simulink model "Pointmass_eom_v1_0"  (R2020a)
settings: Solver=ode4  StartTime=0.0  StopTime=simInit.TSIM  FixedStep=simInit.dt  MaxStep=simInit.dt  RelTol=1e-3
InitFcn:
  | close all
values from neighbouring files (symbols this model uses):
  base_windspeed = 12    [initAllSimParams_DE2019.m]
undefined symbols (not defined in the file or in its folder): constr, DE2019, DiscIntNeverNeededParam, ENVMT, Lbooth, loiterStates, params, simInit, T
libraries: simulink x26, simulink_extras x3
(part 2 of 4)

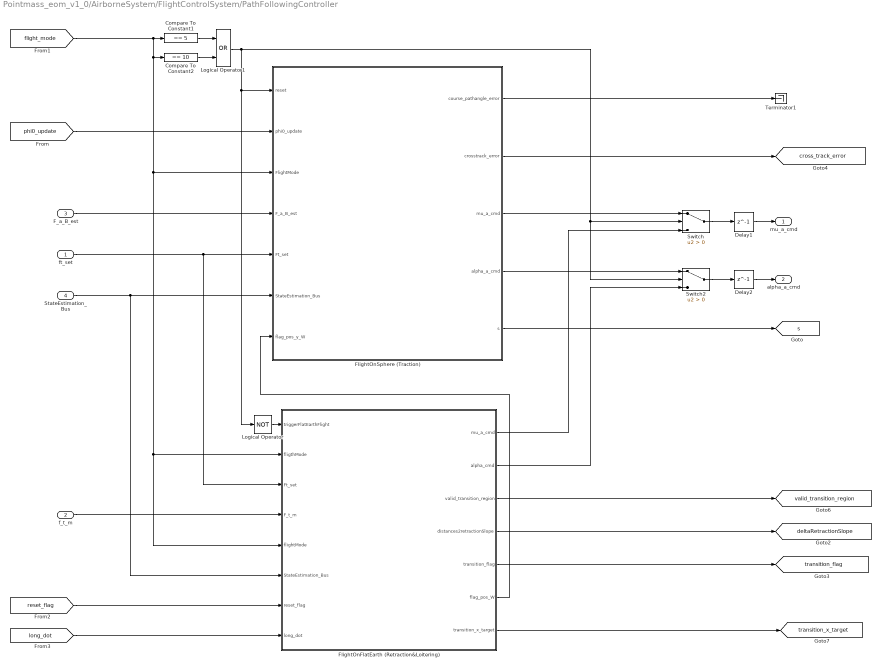
== system Pointmass_eom_v1_0/AirborneSystem/FlightControlSystem/PathFollowingController ==
  ft_set : Inport
  f_t_m : Inport  Port=2
  F_a_B_est : Inport  Port=3  PortDimensions=[3,1]
  StateEstimation_Bus : Inport  Port=4
  Compare To Constant1 : simulink/Logic and Bit Operations/Compare To Constant  relop===  const=5  OutDataTypeStr=boolean
  Compare To Constant2 : simulink/Logic and Bit Operations/Compare To Constant  relop===  const=10  OutDataTypeStr=boolean
  Delay1 : Delay  DelayLength=1
  Delay2 : Delay  DelayLength=1
  FlightOnFlatEarth (Retraction&Loitering) : Subsystem
  FlightOnSphere (Traction) : Subsystem
  Logical Operator : Logic  Operator=NOT  AllPortsSameDT=off  OutDataTypeStr=boolean
  Logical Operator1 : Logic  Operator=OR  AllPortsSameDT=off  OutDataTypeStr=boolean
  Switch : Switch  Criteria=u2 > Threshold
  Switch2 : Switch  Criteria=u2 > Threshold
  Terminator1 : Terminator
  mu_a_cmd : Outport  PortDimensions=1  VectorParamsAs1DForOutWhenUnconnected=off
  alpha_a_cmd : Outport  Port=2  PortDimensions=1  VectorParamsAs1DForOutWhenUnconnected=off
  tag scope: cross_track_error=global, deltaRetractionSlope=global, s=global, transition_flag=global, transition_x_target=global, valid_transition_region=global
  wires:
  StateEstimation_Bus/1 -> FlightOnFlatEarth (Retraction&Loitering)/6(StateEstimation_Bus), FlightOnSphere (Traction)/6(StateEstimation_Bus)
  Logical Operator1/1 -> Switch2/2, Switch/2, FlightOnSphere (Traction)/1(reset), Logical Operator/1
  FlightOnFlatEarth (Retraction&Loitering)/3(valid_transition_region) -> [valid_transition_region]
  FlightOnFlatEarth (Retraction&Loitering)/2(alpha_cmd) -> Switch2/3
  FlightOnFlatEarth (Retraction&Loitering)/1(mu_a_cmd) -> Switch/3
  Logical Operator/1 -> FlightOnFlatEarth (Retraction&Loitering)/1(triggerFlatEarthFlight)
  ft_set/1 -> FlightOnFlatEarth (Retraction&Loitering)/3(Ft_set), FlightOnSphere (Traction)/5(Ft_set)
  Delay2/1 -> alpha_a_cmd/1
  Delay1/1 -> mu_a_cmd/1
  Switch/1 -> Delay1/1
  Switch2/1 -> Delay2/1
  f_t_m/1 -> FlightOnFlatEarth (Retraction&Loitering)/4(F_t_m)
  F_a_B_est/1 -> FlightOnSphere (Traction)/4(F_a_B_est)
  FlightOnSphere (Traction)/4(alpha_a_cmd) -> Switch2/1
  FlightOnSphere (Traction)/3(mu_a_cmd) -> Switch/1
  FlightOnSphere (Traction)/1(course_pathangle_error) -> Terminator1/1
  FlightOnSphere (Traction)/2(crosstrack_error) -> [cross_track_error]
  [flight_mode] -> FlightOnFlatEarth (Retraction&Loitering)/5(flightMode), FlightOnFlatEarth (Retraction&Loitering)/2(fligthMode), FlightOnSphere (Traction)/3(FlightMode), Compare To Constant2/1, Compare To Constant1/1
  Compare To Constant1/1 -> Logical Operator1/1
  Compare To Constant2/1 -> Logical Operator1/2
  FlightOnSphere (Traction)/5(s) -> [s]
  [phi0_update] -> FlightOnSphere (Traction)/2(phi0_update)
  FlightOnFlatEarth (Retraction&Loitering)/5(transition_flag) -> [transition_flag]
  [reset_flag] -> FlightOnFlatEarth (Retraction&Loitering)/7(reset_flag)
  FlightOnFlatEarth (Retraction&Loitering)/4(distances2retractionSlope) -> [deltaRetractionSlope]
  FlightOnFlatEarth (Retraction&Loitering)/6(flag_pos_W) -> FlightOnSphere (Traction)/7(flag_pos_y_W)
  [long_dot] -> FlightOnFlatEarth (Retraction&Loitering)/8(long_dot)
  FlightOnFlatEarth (Retraction&Loitering)/7(transition_x_target) -> [transition_x_target]

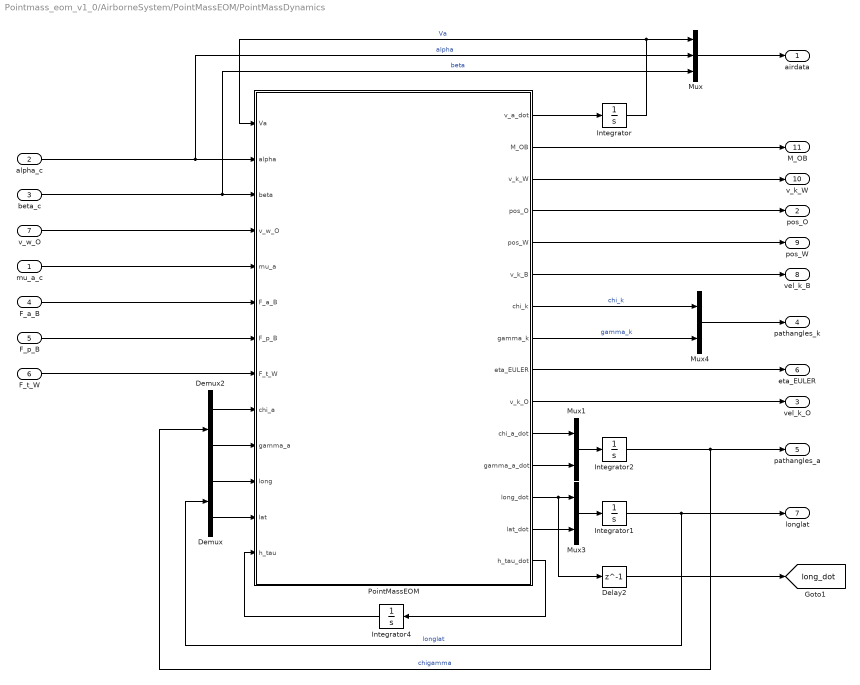
== system Pointmass_eom_v1_0/AirborneSystem/PointMassEOM/PointMassDynamics ==
  mu_a_c : Inport
  alpha_c : Inport  Port=2
  beta_c : Inport  Port=3
  F_a_B : Inport  Port=4  PortDimensions=[3,1]
  F_p_B : Inport  Port=5  PortDimensions=[3,1]
  F_t_W : Inport  Port=6  PortDimensions=[3,1]
  v_w_O : Inport  Port=7
  Delay2 : Delay  DelayLength=1
  Demux : Demux  Outputs=2
  Demux2 : Demux  Outputs=2
  Integrator : Integrator  InitialCondition=.7*loiterStates.Va_set
  Integrator1 : Integrator  InitialCondition=[simInit.long_init;simInit.lat_init]  WrapState=on
  Integrator2 : Integrator  WrapState=on
  Integrator4 : Integrator  InitialCondition=norm(simInit.pos_O_init)
  Mux : Mux  Inputs=3
  Mux1 : Mux  Inputs=2
  Mux3 : Mux  Inputs=2
  Mux4 : Mux  Inputs=2
  PointMassEOM : MATLAB Function  TreatAsAtomicUnit=on
  airdata : Outport  PortDimensions=3  VectorParamsAs1DForOutWhenUnconnected=off
  pos_O : Outport  Port=2  PortDimensions=[3,1]  VectorParamsAs1DForOutWhenUnconnected=off
  vel_k_O : Outport  Port=3  PortDimensions=[3,1]  VectorParamsAs1DForOutWhenUnconnected=off
  pathangles_k : Outport  Port=4  PortDimensions=2  VectorParamsAs1DForOutWhenUnconnected=off
  pathangles_a : Outport  Port=5  PortDimensions=2  VectorParamsAs1DForOutWhenUnconnected=off
  eta_EULER : Outport  Port=6  PortDimensions=[3,1]  VectorParamsAs1DForOutWhenUnconnected=off
  longlat : Outport  Port=7  PortDimensions=2  VectorParamsAs1DForOutWhenUnconnected=off
  vel_k_B : Outport  Port=8  PortDimensions=[3,1]  VectorParamsAs1DForOutWhenUnconnected=off
  pos_W : Outport  Port=9  PortDimensions=[3,1]  VectorParamsAs1DForOutWhenUnconnected=off
  v_k_W : Outport  Port=10  PortDimensions=[3,1]  VectorParamsAs1DForOutWhenUnconnected=off
  M_OB : Outport  Port=11  PortDimensions=[3,3]  VectorParamsAs1DForOutWhenUnconnected=off
  tag scope: long_dot=global
  wires:
  F_p_B/1 -> PointMassEOM/7(F_p_B)
  mu_a_c/1 -> PointMassEOM/5(mu_a)
  PointMassEOM/7(chi_k) -> Mux4/1  "chi_k"
  F_a_B/1 -> PointMassEOM/6(F_a_B)
  Integrator/1 -> PointMassEOM/1(Va), Mux/1  "Va"
  PointMassEOM/8(gamma_k) -> Mux4/2  "gamma_k"
  PointMassEOM/12(gamma_a_dot) -> Mux1/2
  Integrator4/1 -> PointMassEOM/13(h_tau)
  PointMassEOM/14(lat_dot) -> Mux3/2
  PointMassEOM/11(chi_a_dot) -> Mux1/1
  PointMassEOM/15(h_tau_dot) -> Integrator4/1
  PointMassEOM/1(v_a_dot) -> Integrator/1
  Demux2/2 -> PointMassEOM/10(gamma_a)
  v_w_O/1 -> PointMassEOM/4(v_w_O)
  PointMassEOM/9(eta_EULER) -> eta_EULER/1
  Mux/1 -> airdata/1
  alpha_c/1 -> PointMassEOM/2(alpha), Mux/2  "alpha"
  beta_c/1 -> Mux/3, PointMassEOM/3(beta)  "beta"
  PointMassEOM/10(v_k_O) -> vel_k_O/1
  PointMassEOM/6(v_k_B) -> vel_k_B/1
  PointMassEOM/5(pos_W) -> pos_W/1
  PointMassEOM/4(pos_O) -> pos_O/1
  Mux4/1 -> pathangles_k/1
  Demux2/1 -> PointMassEOM/9(chi_a)
  PointMassEOM/3(v_k_W) -> v_k_W/1
  PointMassEOM/2(M_OB) -> M_OB/1
  PointMassEOM/13(long_dot) -> Mux3/1, Delay2/1
  Mux3/1 -> Integrator1/1
  Delay2/1 -> [long_dot]
  Integrator1/1 -> longlat/1, Demux/1  "longlat"
  Demux/1 -> PointMassEOM/11(long)
  Demux/2 -> PointMassEOM/12(lat)
  Mux1/1 -> Integrator2/1
  Integrator2/1 -> pathangles_a/1, Demux2/1  "chigamma"
  F_t_W/1 -> PointMassEOM/8(F_t_W)

== system Pointmass_eom_v1_0/Environment/ShearWind/Length Conversion ==
  in : Inport  Unit=m
  Unit Conversion : UnitConversion
  out : Outport  Unit=ft  VectorParamsAs1DForOutWhenUnconnected=off
  wires:
  in/1 -> Unit Conversion/1
  Unit Conversion/1 -> out/1

== system Pointmass_eom_v1_0/Environment/Windshear/Wind Shear Model ==
  Altitude : Inport  Unit=m
  DCM : Inport  Port=2  Unit=1  PortDimensions=[3 3]
  3ft-->inf1 : Saturate  UpperLimit=inf  LowerLimit=3
  Degrees to Radians : simulink_extras/Transformations/Degrees to Radians
  Disallow CGS : UnitConfiguration  UnitSystemsStr=English,SI,SI (extended)  AllowAllUnitSystems=off
  Length Conversion1 : Subsystem
  Mux : Mux  Inputs=3
  Product2 : Product  Inputs=*/  InputSameDT=on  SaturateOnIntegerOverflow=on  OutDataTypeStr=Inherit: Same as first input
  Product3 : Product  InputSameDT=on  SaturateOnIntegerOverflow=on  OutDataTypeStr=Inherit: Same as first input
  Reshape : Reshape  OutputDimensionality=Column vector (2-D)
  Reshape1 : Reshape
  SinCos : Trigonometry  Operator=sincos
  Transform from Inertial to Body axes : Product  Inputs=**  Multiplication=Matrix(*)  InputSameDT=on  SaturateOnIntegerOverflow=on  OutDataTypeStr=Inherit: Same as first input
  Wdeg1 : Constant  Value=0  OutDataTypeStr=Inherit: Inherit via back propagation
  Wind Direction : Constant  Value=ENVMT.windDirection_rad*180/pi  OutDataTypeStr=Inherit: Inherit via back propagation
  Wind speed at reference height : Gain  Gain=-base_windspeed  SaturateOnIntegerOverflow=on  OutDataTypeStr=Inherit: Same as input  ParamDataTypeStr=Inherit: Same as input
  h/z1 : Gain  Gain=1/0.15  SaturateOnIntegerOverflow=on  OutDataTypeStr=Inherit: Same as input  ParamDataTypeStr=Inherit: Same as input
  ln(h/z0)1 : Math  Operator=log  SignedPower=on  SaturateOnIntegerOverflow=on
  ln(ref_height/z0)1 : Math  Operator=log  SignedPower=on  SaturateOnIntegerOverflow=on
  ref_height/z0 [ft] : Constant  Value=20/0.15  OutDataTypeStr=Inherit: Inherit via back propagation
  Mean Wind : Outport  Unit=m/s  VectorParamsAs1DForOutWhenUnconnected=off
  wires:
  Reshape1/1 -> Mean Wind/1
  Reshape/1 -> Transform from Inertial to Body axes/2
  Degrees to Radians/1 -> SinCos/1
  Wind speed at reference height/1 -> Product3/2
  DCM/1 -> Transform from Inertial to Body axes/1
  Product3/1 -> Reshape/1
  Mux/1 -> Wind speed at reference height/1
  Wdeg1/1 -> Mux/3  "Wz"
  SinCos/1 -> Mux/2  "Wy"
  SinCos/2 -> Mux/1  "Wx"
  Wind Direction/1 -> Degrees to Radians/1
  Transform from Inertial to Body axes/1 -> Reshape1/1
  Altitude/1 -> Length Conversion1/1(in)
  Length Conversion1/1(out) -> 3ft-->inf1/1
  ln(h/z0)1/1 -> Product2/1
  ln(ref_height/z0)1/1 -> Product2/2
  Product2/1 -> Product3/1
  3ft-->inf1/1 -> h/z1/1
  ref_height/z0 [ft]/1 -> ln(ref_height/z0)1/1
  h/z1/1 -> ln(h/z0)1/1

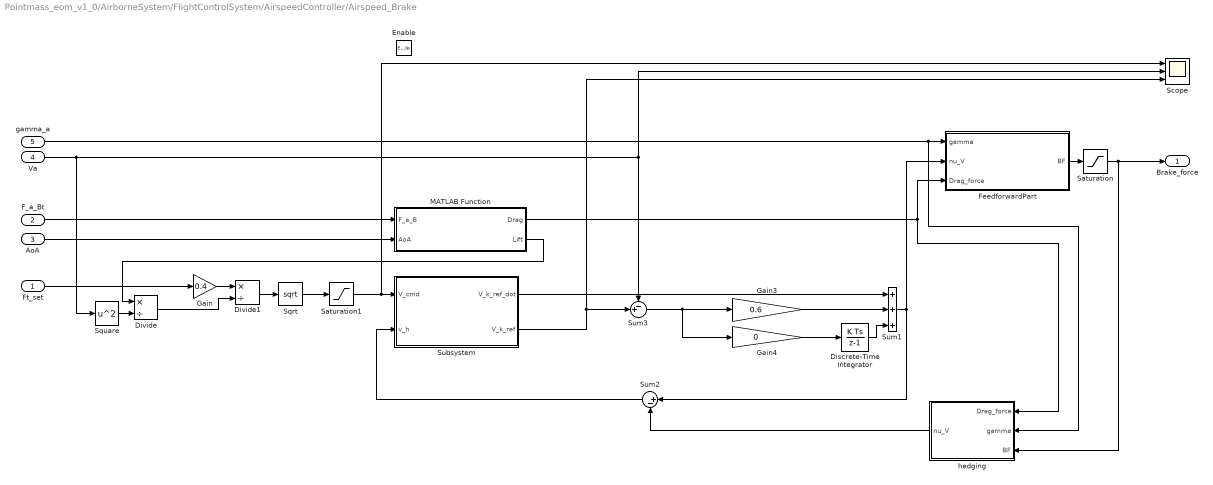
== system Pointmass_eom_v1_0/AirborneSystem/FlightControlSystem/AirspeedController/Airspeed_Brake ==
  Ft_set : Inport
  F_a_Bt : Inport  Port=2  PortDimensions=[3,1]
  AoA : Inport  Port=3
  Va : Inport  Port=4
  gamma_a : Inport  Port=5
  Enable : EnablePort
  Discrete-Time Integrator : DiscreteIntegrator  SampleTime=-1  ICPrevOutput=DiscIntNeverNeededParam  ICPrevScaledInput=DiscIntNeverNeededParam
  Divide : Product  Inputs=*/
  Divide1 : Product  Inputs=*/
  FeedforwardPart : MATLAB Function  TreatAsAtomicUnit=on
  Gain : Gain  Gain=0.4
  Gain3 : Gain  Gain=0.6
  Gain4 : Gain  Gain=0
  MATLAB Function : MATLAB Function  TreatAsAtomicUnit=on
  Saturation : Saturate  UpperLimit=0  LowerLimit=-inf  LinearizeAsGain=off
  Saturation1 : Saturate  UpperLimit=inf  LowerLimit=35
  Scope : Scope  NumInputPorts=3
  Sqrt : Sqrt  SaturateOnIntegerOverflow=on
  Square : Math  Operator=square  SaturateOnIntegerOverflow=on
  Subsystem : Subsystem
  Sum1 : Sum  Inputs=+++
  Sum2 : Sum  Inputs=|+-
  Sum3 : Sum  Inputs=-+|
  hedging : MATLAB Function  TreatAsAtomicUnit=on
  Brake_force : Outport  VectorParamsAs1DForOutWhenUnconnected=off
  wires:
  AoA/1 -> MATLAB Function/2(AoA)
  MATLAB Function/1(Drag) -> hedging/1(Drag_force), FeedforwardPart/3(Drag_force)
  F_a_Bt/1 -> MATLAB Function/1(F_a_B)
  Sum2/1 -> Subsystem/2(v_h)
  hedging/1(nu_V) -> Sum2/2
  FeedforwardPart/1(BF) -> Saturation/1
  Saturation/1 -> hedging/3(BF), Brake_force/1
  Subsystem/1(V_k_ref_dot) -> Sum1/1
  Sum1/1 -> FeedforwardPart/2(nu_V), Sum2/1
  Subsystem/2(V_k_ref) -> Sum3/2, Scope/3
  gamma_a/1 -> hedging/2(gamma), FeedforwardPart/1(gamma)
  Sqrt/1 -> Saturation1/1
  Sum3/1 -> Gain4/1, Gain3/1
  Gain3/1 -> Sum1/2
  Discrete-Time Integrator/1 -> Sum1/3
  Gain4/1 -> Discrete-Time Integrator/1
  MATLAB Function/2(Lift) -> Divide/1
  Va/1 -> Sum3/1, Scope/2, Square/1
  Square/1 -> Divide/2
  Ft_set/1 -> Gain/1
  Divide/1 -> Divide1/2
  Divide1/1 -> Sqrt/1
  Gain/1 -> Divide1/1
  Saturation1/1 -> Subsystem/1(V_cmd), Scope/1

== system Pointmass_eom_v1_0/AirborneSystem/FlightControlSystem/AirspeedController/Airspeed_Control ==
  V_CMD : Inport
  F_a_B : Inport  Port=2  PortDimensions=[3,1]
  AoA : Inport  Port=3
  Va : Inport  Port=4
  gamma_a : Inport  Port=5
  Enable : EnablePort
  Discrete-Time Integrator : DiscreteIntegrator  SampleTime=-1  ICPrevOutput=DiscIntNeverNeededParam  ICPrevScaledInput=DiscIntNeverNeededParam
  FeedforwardPart : MATLAB Function  TreatAsAtomicUnit=on
  Gain3 : Gain  Gain=params.kp_speed_control
  Gain4 : Gain  Gain=params.ki_speed_control
  MATLAB Function : MATLAB Function  TreatAsAtomicUnit=on
  Saturation : Saturate  UpperLimit=inf  LowerLimit=0  LinearizeAsGain=off
  Scope : Scope  NumInputPorts=3
  Subsystem : Subsystem
  Sum : Sum  Inputs=-+|
  Sum1 : Sum  Inputs=+++
  Sum2 : Sum  Inputs=|+-
  hedging : MATLAB Function  TreatAsAtomicUnit=on
  thrust_force : Outport  VectorParamsAs1DForOutWhenUnconnected=off
  wires:
  AoA/1 -> MATLAB Function/2(AoA)
  MATLAB Function/1(Drag) -> hedging/1(Drag_force), FeedforwardPart/3(Drag_force)
  F_a_B/1 -> MATLAB Function/1(F_a_B)
  Sum2/1 -> Subsystem/2(v_h)
  hedging/1(nu_V) -> Sum2/2
  FeedforwardPart/1(T) -> Saturation/1
  Saturation/1 -> thrust_force/1, hedging/3(T)
  Subsystem/1(V_k_ref_dot) -> Sum1/1
  Sum1/1 -> Sum2/1, FeedforwardPart/2(nu_V)
  Subsystem/2(V_k_ref) -> Sum/2, Scope/3
  gamma_a/1 -> hedging/2(gamma), FeedforwardPart/1(gamma)
  V_CMD/1 -> Subsystem/1(V_cmd), Scope/1
  Sum/1 -> Gain4/1, Gain3/1
  Va/1 -> Scope/2, Sum/1
  Gain3/1 -> Sum1/2
  Discrete-Time Integrator/1 -> Sum1/3
  Gain4/1 -> Discrete-Time Integrator/1

== system Pointmass_eom_v1_0/AirborneSystem/FlightControlSystem/PathFollowingController/FlightOnFlatEarth (Retraction&Loitering) ==
  triggerFlatEarthFlight : Inport
  fligthMode : Inport  Port=2
  Ft_set : Inport  Port=3
  F_t_m : Inport  Port=4
  flightMode : Inport  Port=5
  StateEstimation_Bus : Inport  Port=6
  reset_flag : Inport  Port=7
  long_dot : Inport  Port=8
  CalculateAttitudeCmds : Subsystem
  GuidanceFlatEarth : Subsystem
  mu_a_cmd : Outport  VectorParamsAs1DForOutWhenUnconnected=off
  alpha_cmd : Outport  Port=2  VectorParamsAs1DForOutWhenUnconnected=off
  valid_transition_region : Outport  Port=3  VectorParamsAs1DForOutWhenUnconnected=off
  distances2retractionSlope : Outport  Port=4  VectorParamsAs1DForOutWhenUnconnected=off
  transition_flag : Outport  Port=5  VectorParamsAs1DForOutWhenUnconnected=off
  flag_pos_W : Outport  Port=6  VectorParamsAs1DForOutWhenUnconnected=off
  transition_x_target : Outport  Port=7  VectorParamsAs1DForOutWhenUnconnected=off
  wires:
  StateEstimation_Bus/1 -> GuidanceFlatEarth/2(StateEstimation_Bus), CalculateAttitudeCmds/6(StateEstimation_Bus)
  CalculateAttitudeCmds/1(mu_a_cmd) -> mu_a_cmd/1
  Ft_set/1 -> CalculateAttitudeCmds/3(Ft_set)
  CalculateAttitudeCmds/2(alpha_cmd) -> alpha_cmd/1
  fligthMode/1 -> GuidanceFlatEarth/1(flightMode)
  triggerFlatEarthFlight/1 -> GuidanceFlatEarth/Enable, CalculateAttitudeCmds/1(flight_on_flatearth_flag)
  GuidanceFlatEarth/2(valid_transition_region) -> valid_transition_region/1
  F_t_m/1 -> CalculateAttitudeCmds/4(F_t_m)
  GuidanceFlatEarth/1(distances2slope) -> distances2retractionSlope/1
  GuidanceFlatEarth/3(course_path) -> CalculateAttitudeCmds/2(pathangles_k_cmd)
  flightMode/1 -> CalculateAttitudeCmds/5(flightMode)
  GuidanceFlatEarth/4(transition_flag) -> transition_flag/1
  reset_flag/1 -> GuidanceFlatEarth/3(reset_flat)
  GuidanceFlatEarth/5(flag_pos_W) -> flag_pos_W/1
  long_dot/1 -> GuidanceFlatEarth/4(long_dot)
  GuidanceFlatEarth/6(transition_x_target) -> transition_x_target/1

== system Pointmass_eom_v1_0/AirborneSystem/FlightControlSystem/PathFollowingController/FlightOnSphere (Traction) ==
  reset : Inport
  phi0_update : Inport  Port=2
  FlightMode : Inport  Port=3  PortDimensions=1
  F_a_B_est : Inport  Port=4  PortDimensions=[3,1]
  Ft_set : Inport  Port=5
  StateEstimation_Bus : Inport  Port=6
  flag_pos_y_W : Inport  Port=7
  Constant : Constant  Value=Lbooth.init_sol
  FlightPathLoopTraction : Subsystem
  Navigator : Subsystem
  Pcontroller_ChiGamma_Traction : Subsystem
  Select_init_sol_for_pathfollowing : Stateflow chart  TreatAsAtomicUnit=on
  Sum : Sum  Inputs=|++
  Sum1 : Sum  Inputs=|++
  course_pathangle_error : Outport  VectorParamsAs1DForOutWhenUnconnected=off
  crosstrack_error : Outport  Port=2  VectorParamsAs1DForOutWhenUnconnected=off
  mu_a_cmd : Outport  Port=3  PortDimensions=1  VectorParamsAs1DForOutWhenUnconnected=off
  alpha_a_cmd : Outport  Port=4  PortDimensions=1  VectorParamsAs1DForOutWhenUnconnected=off
  s : Outport  Port=5  VectorParamsAs1DForOutWhenUnconnected=off
  wires:
  FlightPathLoopTraction/1(mu_a_c_traction) -> mu_a_cmd/1
  Navigator/5(course_pathangle_error) -> Pcontroller_ChiGamma_Traction/1(course_pathangle_error), course_pathangle_error/1
  Navigator/1(crosstrack_error) -> crosstrack_error/1
  FlightPathLoopTraction/2(alpha_rq) -> alpha_a_cmd/1
  F_a_B_est/1 -> FlightPathLoopTraction/2(F_a_B_est)
  Ft_set/1 -> FlightPathLoopTraction/1(Ft_set)
  StateEstimation_Bus/1 -> FlightPathLoopTraction/3(StateEstimation_Bus), Navigator/3(StateEstimation_Bus)
  Navigator/2(s) -> s/1
  phi0_update/1 -> Navigator/1(phi0_update)
  reset/1 -> FlightPathLoopTraction/Enable, Navigator/Enable
  Navigator/3(chi_k_dot) -> Sum/1
  Navigator/4(gamma_k_dot) -> Sum1/1
  Select_init_sol_for_pathfollowing/1(sol_init) -> Navigator/4(init_value)
  Constant/1 -> Select_init_sol_for_pathfollowing/1(x)
  Sum1/1 -> FlightPathLoopTraction/5(nu_gamma)
  Sum/1 -> FlightPathLoopTraction/4(nu_chi)
  FlightMode/1 -> Navigator/2(flight_mode), Select_init_sol_for_pathfollowing/2(fm)
  flag_pos_y_W/1 -> Select_init_sol_for_pathfollowing/3(flag_pos_y_W)
  Pcontroller_ChiGamma_Traction/1(Chi_cntr) -> Sum/2
  Pcontroller_ChiGamma_Traction/2(Gamma_cntr) -> Sum1/2

== system Pointmass_eom_v1_0/Environment/Windshear/Wind Shear Model/Length Conversion1 ==
  in : Inport  Unit=m
  Unit Conversion : UnitConversion
  out : Outport  Unit=ft  VectorParamsAs1DForOutWhenUnconnected=off
  wires:
  in/1 -> Unit Conversion/1
  Unit Conversion/1 -> out/1

== system Pointmass_eom_v1_0/AirborneSystem/FlightControlSystem/AirspeedController/Airspeed_Brake/Subsystem ==
  V_cmd : Inport
  v_h : Inport  Port=2
  Discrete-Time Integrator1 : DiscreteIntegrator  InitialCondition=norm(simInit.vel_B_init)  SampleTime=-1  LimitOutput=on  UpperSaturationLimit=120  LowerSaturationLimit=0  ICPrevOutput=DiscIntNeverNeededParam  ICPrevScaledInput=DiscIntNeverNeededParam
  Gain2 : Gain  Gain=params.w0SpeedControl  Multiplication=Matrix(K*u)
  Sum1 : Sum  Inputs=|+-
  Sum2 : Sum  Inputs=|+-
  V_k_ref_dot : Outport  VectorParamsAs1DForOutWhenUnconnected=off
  V_k_ref : Outport  Port=2  VectorParamsAs1DForOutWhenUnconnected=off
  wires:
  Gain2/1 -> Sum1/1, V_k_ref_dot/1
  v_h/1 -> Sum1/2
  Sum1/1 -> Discrete-Time Integrator1/1
  V_cmd/1 -> Sum2/1
  Sum2/1 -> Gain2/1
  Discrete-Time Integrator1/1 -> V_k_ref/1, Sum2/2

== system Pointmass_eom_v1_0/AirborneSystem/FlightControlSystem/AirspeedController/Airspeed_Control/Subsystem ==
  V_cmd : Inport
  v_h : Inport  Port=2
  Discrete-Time Integrator1 : DiscreteIntegrator  InitialCondition=norm(simInit.vel_B_init)  SampleTime=-1  LimitOutput=on  UpperSaturationLimit=120  LowerSaturationLimit=0  ICPrevOutput=DiscIntNeverNeededParam  ICPrevScaledInput=DiscIntNeverNeededParam
  Gain2 : Gain  Gain=params.w0SpeedControl  Multiplication=Matrix(K*u)
  Sum1 : Sum  Inputs=|+-
  Sum2 : Sum  Inputs=|+-
  V_k_ref_dot : Outport  VectorParamsAs1DForOutWhenUnconnected=off
  V_k_ref : Outport  Port=2  VectorParamsAs1DForOutWhenUnconnected=off
  wires:
  Gain2/1 -> Sum1/1, V_k_ref_dot/1
  v_h/1 -> Sum1/2
  Sum1/1 -> Discrete-Time Integrator1/1
  V_cmd/1 -> Sum2/1
  Sum2/1 -> Gain2/1
  Discrete-Time Integrator1/1 -> V_k_ref/1, Sum2/2

== system Pointmass_eom_v1_0/AirborneSystem/FlightControlSystem/PathFollowingController/FlightOnFlatEarth (Retraction&Loitering)/CalculateAttitudeCmds ==
  flight_on_flatearth_flag : Inport
  pathangles_k_cmd : Inport  Port=2
  Ft_set : Inport  Port=3
  F_t_m : Inport  Port=4
  flightMode : Inport  Port=5
  StateEstimation_Bus : Inport  Port=6
  Demux : Demux  Outputs=3
  FlightPathLoopRetraction_Aerodynamic : Subsystem
  Mux1 : Mux  Inputs=3
  Signal Specification : SignalSpecification  Dimensions=[3,1]
  Terminator2 : Terminator
  mu_a_cmd : Outport  VectorParamsAs1DForOutWhenUnconnected=off
  alpha_cmd : Outport  Port=2  VectorParamsAs1DForOutWhenUnconnected=off
  wires:
  StateEstimation_Bus/1 -> FlightPathLoopRetraction_Aerodynamic/4(StateEstimation_Bus)
  Demux/3 -> Terminator2/1
  Demux/2 -> alpha_cmd/1
  flight_on_flatearth_flag/1 -> FlightPathLoopRetraction_Aerodynamic/Enable
  FlightPathLoopRetraction_Aerodynamic/2(alpha_a_cmd) -> Mux1/2
  flightMode/1 -> FlightPathLoopRetraction_Aerodynamic/1(flight_mode)
  Signal Specification/1 -> Demux/1
  Demux/1 -> mu_a_cmd/1
  Mux1/1 -> Signal Specification/1
  F_t_m/1 -> FlightPathLoopRetraction_Aerodynamic/3(F_t_m)
  FlightPathLoopRetraction_Aerodynamic/1(mu_a_cmd) -> Mux1/1
  Ft_set/1 -> FlightPathLoopRetraction_Aerodynamic/2(F_t_set)
  FlightPathLoopRetraction_Aerodynamic/3(beta_a_cmd) -> Mux1/3
  pathangles_k_cmd/1 -> FlightPathLoopRetraction_Aerodynamic/5(kinematic_path_cmd)

== system Pointmass_eom_v1_0/AirborneSystem/FlightControlSystem/PathFollowingController/FlightOnFlatEarth (Retraction&Loitering)/GuidanceFlatEarth ==
  flightMode : Inport
  StateEstimation_Bus : Inport  Port=2
  reset_flat : Inport  Port=3
  long_dot : Inport  Port=4
  Enable : EnablePort
  Bus Selector : BusSelector  OutputSignals=pos_G_O_m,vel_K_O_mDs,pathangles_k,pos_G_W
  Compare To Constant : simulink/Logic and Bit Operations/Compare To Constant  relop===  const=6  OutDataTypeStr=boolean
  Compare To Constant2 : simulink/Logic and Bit Operations/Compare To Constant  relop===  const=6  OutDataTypeStr=boolean
  LoiteringGuidance : Subsystem
  Retraction_Nav : Subsystem
  Switch1 : Switch  Criteria=u2 > Threshold
  distances2slope : Outport  VectorParamsAs1DForOutWhenUnconnected=off
  valid_transition_region : Outport  Port=2  VectorParamsAs1DForOutWhenUnconnected=off
  course_path : Outport  Port=3  VectorParamsAs1DForOutWhenUnconnected=off
  transition_flag : Outport  Port=4  VectorParamsAs1DForOutWhenUnconnected=off
  flag_pos_W : Outport  Port=5  VectorParamsAs1DForOutWhenUnconnected=off
  transition_x_target : Outport  Port=6  VectorParamsAs1DForOutWhenUnconnected=off
  wires:
  Bus Selector/1 -> LoiteringGuidance/2(<pos_G_O_m>), Retraction_Nav/2(pos_O)  "<pos_G_O_m>"
  StateEstimation_Bus/1 -> Bus Selector/1
  Bus Selector/2 -> LoiteringGuidance/3(<vel_K_O_mDs>), Retraction_Nav/3(vel_k_O)  "<vel_K_O_mDs>"
  Compare To Constant2/1 -> Retraction_Nav/Enable
  Switch1/1 -> course_path/1
  Compare To Constant/1 -> Switch1/2
  Retraction_Nav/1(distances2slope) -> distances2slope/1
  Retraction_Nav/2(path_k_cmds) -> Switch1/1
  flightMode/1 -> Retraction_Nav/1(flight_mode), Compare To Constant/1, LoiteringGuidance/1(flightMode), Compare To Constant2/1
  Bus Selector/3 -> LoiteringGuidance/4(<pathangles_k>)  "<pathangles_k>"
  LoiteringGuidance/1(path_k_cmds) -> Switch1/3
  LoiteringGuidance/2(valid_transition_region) -> valid_transition_region/1
  Retraction_Nav/3(transition_flag) -> transition_flag/1
  reset_flat/1 -> LoiteringGuidance/6(reset_flag)
  Bus Selector/4 -> LoiteringGuidance/5(pos_W)  "<pos_G_W>"
  Retraction_Nav/4(flag_pos_y_W) -> flag_pos_W/1
  long_dot/1 -> Retraction_Nav/4(long_dot)
  Retraction_Nav/5(transition_x_target) -> transition_x_target/1

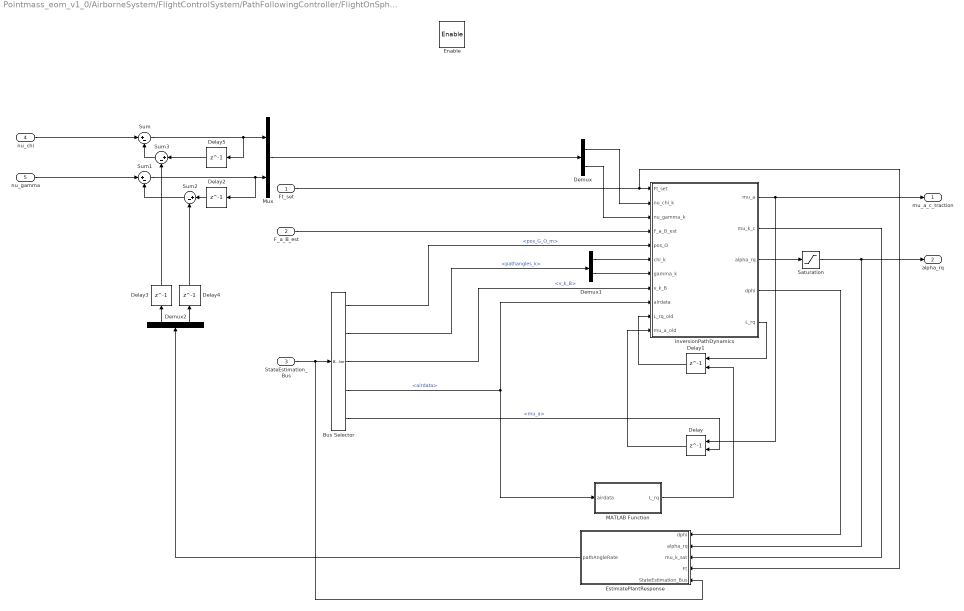
== system Pointmass_eom_v1_0/AirborneSystem/FlightControlSystem/PathFollowingController/FlightOnSphere (Traction)/FlightPathLoopTraction ==
  Ft_set : Inport
  F_a_B_est : Inport  Port=2  PortDimensions=[3,1]
  StateEstimation_Bus : Inport  Port=3
  nu_chi : Inport  Port=4
  nu_gamma : Inport  Port=5
  Enable : EnablePort  StatesWhenEnabling=reset
  Bus Selector : BusSelector  OutputSignals=pos_G_O_m,pathangles_k,v_k_B,airdata,mu_a
  Delay : Delay  DelayLength=1  InitialConditionSource=Input port
      settings: InputPortMap=u0,p4
  Delay1 : Delay  DelayLength=1  InitialConditionSource=Input port
      settings: InputPortMap=u0,p4
  Delay{2..5} (4 alike) : Delay  DelayLength=1
  Demux : Demux  Outputs=2
  Demux1 : Demux  Outputs=2
  Demux2 : Demux  Outputs=2
  EstimatePlantResponse : Subsystem
  MATLAB Function : MATLAB Function  TreatAsAtomicUnit=on
  Mux : Mux  Inputs=2
  Saturation : Saturate  UpperLimit=constr.alpha_a_max  LowerLimit=constr.alpha_a_min
  Sum{,1..3} (4 alike) : Sum  Inputs=|+-
  inversionPathDynamics : MATLAB Function  TreatAsAtomicUnit=on
  mu_a_c_traction : Outport  PortDimensions=1  VectorParamsAs1DForOutWhenUnconnected=off
  alpha_rq : Outport  Port=2  PortDimensions=1  VectorParamsAs1DForOutWhenUnconnected=off
  wires:
  Bus Selector/5 -> Delay/2  "<mu_a>"
  F_a_B_est/1 -> inversionPathDynamics/4(F_a_B_est)
  Demux1/1 -> inversionPathDynamics/6(chi_k)
  inversionPathDynamics/1(mu_a) -> Delay/1, mu_a_c_traction/1
  Mux/1 -> Demux/1
  Demux/2 -> inversionPathDynamics/3(nu_gamma_k)
  Demux/1 -> inversionPathDynamics/2(nu_chi_k)
  inversionPathDynamics/2(mu_k_c) -> EstimatePlantResponse/3(mu_k_sat)
  inversionPathDynamics/3(alpha_rq) -> Saturation/1
  Saturation/1 -> alpha_rq/1, EstimatePlantResponse/2(alpha_rq)
  inversionPathDynamics/4(dphi) -> EstimatePlantResponse/1(dphi)
  Delay1/1 -> inversionPathDynamics/10(L_rq_old)
  Delay/1 -> inversionPathDynamics/11(mu_a_old)
  MATLAB Function/1(L_rq) -> Delay1/2
  inversionPathDynamics/5(L_rq) -> Delay1/1
  Demux1/2 -> inversionPathDynamics/7(gamma_k)
  StateEstimation_Bus/1 -> Bus Selector/1, EstimatePlantResponse/5(StateEstimation_Bus)
  Bus Selector/4 -> inversionPathDynamics/9(airdata), MATLAB Function/1(airdata)  "<airdata>"
  Bus Selector/2 -> Demux1/1  "<pathangles_k>"
  Bus Selector/3 -> inversionPathDynamics/8(v_k_B)  "<v_k_B>"
  Bus Selector/1 -> inversionPathDynamics/5(pos_O)  "<pos_G_O_m>"
  Delay5/1 -> Sum3/1
  nu_chi/1 -> Sum/1
  Sum3/1 -> Sum/2
  Delay4/1 -> Sum2/2
  Delay3/1 -> Sum3/2
  Demux2/2 -> Delay4/1
  Sum1/1 -> Delay2/1, Mux/2
  Sum/1 -> Delay5/1, Mux/1
  Delay2/1 -> Sum2/1
  EstimatePlantResponse/1(pathAngleRate) -> Demux2/1
  nu_gamma/1 -> Sum1/1
  Demux2/1 -> Delay3/1
  Sum2/1 -> Sum1/2
  Ft_set/1 -> inversionPathDynamics/1(Ft_set), EstimatePlantResponse/4(Ft)

== system Pointmass_eom_v1_0/AirborneSystem/FlightControlSystem/PathFollowingController/FlightOnSphere (Traction)/Navigator ==
  phi0_update : Inport
  flight_mode : Inport  Port=2
  StateEstimation_Bus : Inport  Port=3
  init_value : Inport  Port=4
  Enable : EnablePort  StatesWhenEnabling=reset
  Bus Selector : BusSelector  OutputSignals=pathangles_k,pos_G_W,vel_W,vel_K_O_mDs,longlat
  Compare To Constant3 : simulink/Logic and Bit Operations/Compare To Constant  relop===  const=5  OutDataTypeStr=boolean
  Constant : Constant  Value=0
  Constant1 : Constant  Value=0
  Delay1 : Delay  DelayLength=1  InitialConditionSource=Input port  InitialCondition=pi/2  ExternalReset=Rising
      settings: InputPortMap=u0,r5,p4
  Demux : Demux  Outputs=2
  Demux2 : Demux  Outputs=2
  LissajousFigure8Following : MATLAB Function  TreatAsAtomicUnit=on
  Mux : Mux  Inputs=2
  Mux1 : Mux  Inputs=2
  Mux3 : Mux  Inputs=2
  Scope1 : Scope  NumInputPorts=2
  Sum : Sum  Inputs=|+-
  calcualteCourseErrorAndWrap1 : MATLAB Function  TreatAsAtomicUnit=on
  crosstrack_error : Outport  VectorParamsAs1DForOutWhenUnconnected=off
  s : Outport  Port=2  PortDimensions=1  InitialOutput=0  VectorParamsAs1DForOutWhenUnconnected=off
  chi_k_dot : Outport  Port=3  PortDimensions=1  VectorParamsAs1DForOutWhenUnconnected=off
  gamma_k_dot : Outport  Port=4  PortDimensions=1  VectorParamsAs1DForOutWhenUnconnected=off
  course_pathangle_error : Outport  Port=5  VectorParamsAs1DForOutWhenUnconnected=off
  wires:
  Mux3/1 -> Scope1/2
  Mux1/1 -> Scope1/1
  Delay1/1 -> LissajousFigure8Following/10(sol_old)
  LissajousFigure8Following/6(sol) -> Delay1/1, s/1
  Bus Selector/4 -> LissajousFigure8Following/4(v_O_vec)  "<vel_K_O_mDs>"
  Demux/1 -> LissajousFigure8Following/5(long)
  calcualteCourseErrorAndWrap1/1(e_course) -> Mux/1
  LissajousFigure8Following/1(chi_k_ideal) -> calcualteCourseErrorAndWrap1/1(chi_ref), Mux1/1
  LissajousFigure8Following/2(gamma_k_ideal) -> Sum/1, Mux3/1
  Demux2/1 -> Mux1/2, calcualteCourseErrorAndWrap1/2(chi)
  Demux2/2 -> Mux3/2, Sum/2
  Mux/1 -> course_pathangle_error/1
  LissajousFigure8Following/4(gamma_dot) -> gamma_k_dot/1
  LissajousFigure8Following/3(chi_dot) -> chi_k_dot/1
  Sum/1 -> Mux/2
  Demux/2 -> LissajousFigure8Following/6(lat)
  LissajousFigure8Following/5(delta_ct) -> crosstrack_error/1
  StateEstimation_Bus/1 -> Bus Selector/1
  Bus Selector/2 -> LissajousFigure8Following/2(pos_W)  "<pos_G_W>"
  Bus Selector/5 -> Demux/1  "<longlat>"
  Bus Selector/1 -> LissajousFigure8Following/1(pathAngles), Demux2/1  "<pathangles_k>"
  flight_mode/1 -> Compare To Constant3/1
  phi0_update/1 -> LissajousFigure8Following/9(PHI_BOOTH)
  Compare To Constant3/1 -> Delay1/2
  init_value/1 -> Delay1/3
  Constant/1 -> LissajousFigure8Following/7(gamma_tau_dot)
  Bus Selector/3 -> LissajousFigure8Following/3(v_w_vec)  "<vel_W>"
  Constant1/1 -> LissajousFigure8Following/8(gamma_tau_cmd)

== system Pointmass_eom_v1_0/AirborneSystem/FlightControlSystem/PathFollowingController/FlightOnSphere (Traction)/Pcontroller_ChiGamma_Traction ==
  course_pathangle_error : Inport
  Demux : Demux  Outputs=2
  Kp : Gain  Gain=params.Kp_gamma_k_traction  Multiplication=Matrix(K*u)
  Kp1 : Gain  Gain=params.Kp_chi_k_traction  Multiplication=Matrix(K*u)
  Chi_cntr : Outport
  Gamma_cntr : Outport  Port=2
  wires:
  Kp1/1 -> Chi_cntr/1
  Kp/1 -> Gamma_cntr/1
  course_pathangle_error/1 -> Demux/1
  Demux/2 -> Kp/1
  Demux/1 -> Kp1/1

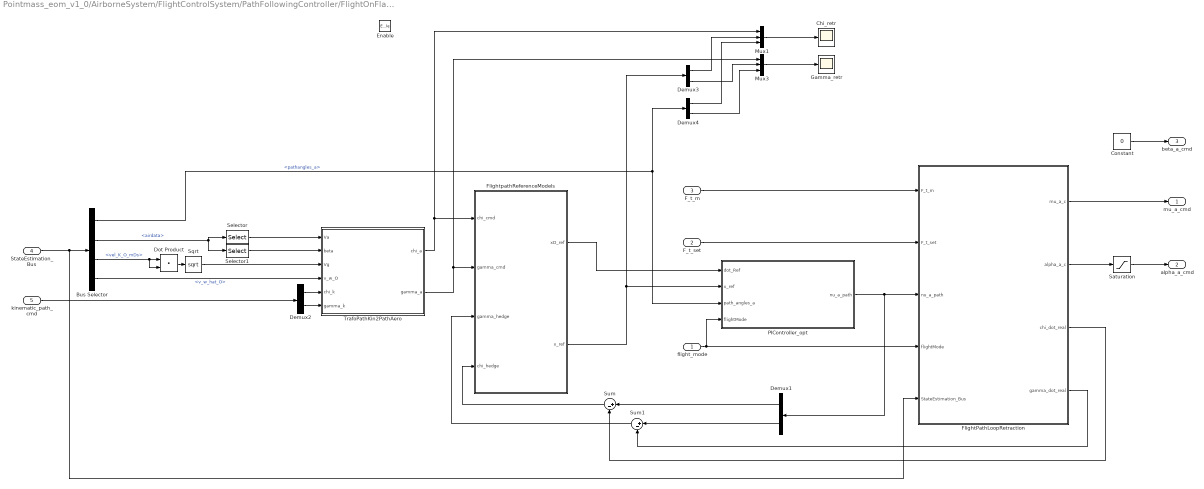
== system Pointmass_eom_v1_0/AirborneSystem/FlightControlSystem/PathFollowingController/FlightOnFlatEarth (Retraction&Loitering)/CalculateAttitudeCmds/FlightPathLoopRetraction_Aerodynamic ==
  flight_mode : Inport
  F_t_set : Inport  Port=2
  F_t_m : Inport  Port=3
  StateEstimation_Bus : Inport  Port=4
  kinematic_path_cmd : Inport  Port=5
  Enable : EnablePort  StatesWhenEnabling=reset
  Bus Selector : BusSelector  OutputSignals=pathangles_a,airdata,vel_K_O_mDs,v_w_hat_O
  Chi_retr : Scope
  Constant : Constant  Value=0
  Demux{1..4} (4 alike) : Demux  Outputs=2
  Dot Product : DotProduct  InputSameDT=on  OutDataTypeStr=Inherit: Inherit via internal rule
  FlightPathLoopRetraction : Subsystem
  FlightpathReferenceModels : Subsystem
  Gamma_retr : Scope
  Mux1 : Mux  Inputs=3
  Mux3 : Mux  Inputs=3
  PIController_opt : Subsystem
  Saturation : Saturate  UpperLimit=constr.alpha_a_max  LowerLimit=constr.alpha_a_min
  Selector : Selector  InputPortWidth=3  IndexOptions=Index vector (dialog)  Indices=1  OutputSizes=1
  Selector1 : Selector  InputPortWidth=3  IndexOptions=Index vector (dialog)  Indices=3  OutputSizes=1
  Sqrt : Sqrt  SaturateOnIntegerOverflow=on
  Sum : Sum  Inputs=|+-
  Sum1 : Sum  Inputs=|+-
  TrafoPathKin2PathAero : MATLAB Function  TreatAsAtomicUnit=on
  mu_a_cmd : Outport  VectorParamsAs1DForOutWhenUnconnected=off
  alpha_a_cmd : Outport  Port=2  VectorParamsAs1DForOutWhenUnconnected=off
  beta_a_cmd : Outport  Port=3  VectorParamsAs1DForOutWhenUnconnected=off
  wires:
  StateEstimation_Bus/1 -> Bus Selector/1, FlightPathLoopRetraction/5(StateEstimation_Bus)
  Bus Selector/1 -> Demux4/1, PIController_opt/3(path_angles_a)  "<pathangles_a>"
  Bus Selector/3 -> Dot Product/2, Dot Product/1  "<vel_K_O_mDs>"
  Bus Selector/2 -> Selector1/1, Selector/1  "<airdata>"
  F_t_m/1 -> FlightPathLoopRetraction/1(F_t_m)
  Sum/1 -> FlightpathReferenceModels/4(chi_hedge)
  Mux3/1 -> Gamma_retr/1
  Mux1/1 -> Chi_retr/1
  Demux4/1 -> Mux1/3
  Demux3/2 -> Mux3/2
  Demux4/2 -> Mux3/3
  Demux3/1 -> Mux1/2
  Demux2/2 -> TrafoPathKin2PathAero/6(gamma_k)
  FlightpathReferenceModels/2(x_ref) -> Demux3/1, PIController_opt/2(x_ref)
  Demux2/1 -> TrafoPathKin2PathAero/5(chi_k)
  FlightPathLoopRetraction/1(mu_a_c) -> mu_a_cmd/1
  FlightpathReferenceModels/1(xD_ref) -> PIController_opt/1(dot_Ref)
  Constant/1 -> beta_a_cmd/1
  Demux1/1 -> Sum/1
  Demux1/2 -> Sum1/1
  FlightPathLoopRetraction/3(chi_dot_real) -> Sum/2
  Sum1/1 -> FlightpathReferenceModels/3(gamma_hedge)
  PIController_opt/1(nu_a_path) -> FlightPathLoopRetraction/3(nu_a_path), Demux1/1
  Saturation/1 -> alpha_a_cmd/1
  FlightPathLoopRetraction/2(alpha_a_c) -> Saturation/1
  Dot Product/1 -> Sqrt/1
  Sqrt/1 -> TrafoPathKin2PathAero/3(Vg)
  Selector/1 -> TrafoPathKin2PathAero/1(Va)
  TrafoPathKin2PathAero/1(chi_a) -> Mux1/1, FlightpathReferenceModels/1(chi_cmd)
  TrafoPathKin2PathAero/2(gamma_a) -> Mux3/1, FlightpathReferenceModels/2(gamma_cmd)
  Selector1/1 -> TrafoPathKin2PathAero/2(beta)
  F_t_set/1 -> FlightPathLoopRetraction/2(F_t_set)
  kinematic_path_cmd/1 -> Demux2/1
  Bus Selector/4 -> TrafoPathKin2PathAero/4(v_w_O)  "<v_w_hat_O>"
  flight_mode/1 -> FlightPathLoopRetraction/4(flightMode), PIController_opt/4(flightMode)
  FlightPathLoopRetraction/4(gamma_dot_real) -> Sum1/2

== system Pointmass_eom_v1_0/AirborneSystem/FlightControlSystem/PathFollowingController/FlightOnFlatEarth (Retraction&Loitering)/GuidanceFlatEarth/LoiteringGuidance ==
  flightMode : Inport
  <pos_G_O_m> : Inport  Port=2
  <vel_K_O_mDs> : Inport  Port=3
  <pathangles_k> : Inport  Port=4
  pos_W : Inport  Port=5
  reset_flag : Inport  Port=6
  Compare To Constant3 : simulink/Logic and Bit Operations/Compare To Constant  relop===  const=1  OutDataTypeStr=boolean
  Constant1 : Constant  Value=ENVMT.windDirection_rad
  Constant3 : Constant  Value=0
  Delay : Delay  DelayLength=1  InitialConditionSource=Input port  ExternalReset=Rising
      settings: InputPortMap=u0,r5,p4
  Delay1 : Delay  DelayLength=1  InitialConditionSource=Input port  ExternalReset=Rising
      settings: InputPortMap=u0,r5,p4
  Dot Product : DotProduct  InputSameDT=on  OutDataTypeStr=Inherit: Inherit via internal rule
  Gain1 : Gain  Gain=-1
  Loiter : Stateflow chart  TreatAsAtomicUnit=on  mask{kp_course_init=params.kp_delta_course, pos_OLoiter_W=loiterStates.pos_OLoiter_W, R_init_loiter=loiterStates.R, validTransReg_start=loiterStates.validTransReg_start, validTransReg_end=loiterStates.validTransReg_end}
  Mux : Mux  Inputs=2
  Selector1 : Selector  InputPortWidth=2  IndexOptions=Index vector (dialog)  Indices=1  OutputSizes=1
  Selector2 : Selector  InputPortWidth=3  IndexOptions=Index vector (dialog)  Indices=2  OutputSizes=1
  Selector3 : Selector  InputPortWidth=3  IndexOptions=Index vector (dialog)  Indices=1  OutputSizes=1
  Selector4 : Selector  InputPortWidth=3  IndexOptions=Index vector (dialog)  Indices=3  OutputSizes=1
  Sqrt : Sqrt  SaturateOnIntegerOverflow=on
  Subsystem : Subsystem
  Terminator1 : Terminator
  path_k_cmds : Outport  VectorParamsAs1DForOutWhenUnconnected=off
  valid_transition_region : Outport  Port=2  VectorParamsAs1DForOutWhenUnconnected=off
  wires:
  <pathangles_k>/1 -> Selector1/1
  Mux/1 -> path_k_cmds/1
  Selector1/1 -> Delay/3
  Selector4/1 -> Gain1/1
  Compare To Constant3/1 -> Delay1/2
  pos_W/1 -> Selector2/1, Selector3/1
  Dot Product/1 -> Sqrt/1
  Sqrt/1 -> Loiter/4(Vk)
  Delay1/1 -> Delay1/1, Subsystem/2(h_cmd)
  Loiter/1(course_des) -> Mux/1
  <vel_K_O_mDs>/1 -> Dot Product/2, Dot Product/1, Subsystem/1(v_k_O)
  <pos_G_O_m>/1 -> Subsystem/3(h), Selector4/1
  Selector3/1 -> Loiter/3(p_x_W)
  Gain1/1 -> Delay1/3
  Subsystem/1(gamma_k_cmd) -> Mux/2
  Delay/1 -> Loiter/2(course_k), Delay/1
  Selector2/1 -> Loiter/1(p_y_W)
  Loiter/2(valid_transition_region_flag) -> valid_transition_region/1
  reset_flag/1 -> Loiter/5(reset_flag)
  Constant1/1 -> Loiter/6(windDir)
  Constant3/1 -> Delay/2
  flightMode/1 -> Compare To Constant3/1
  Loiter/3(e_track) -> Terminator1/1

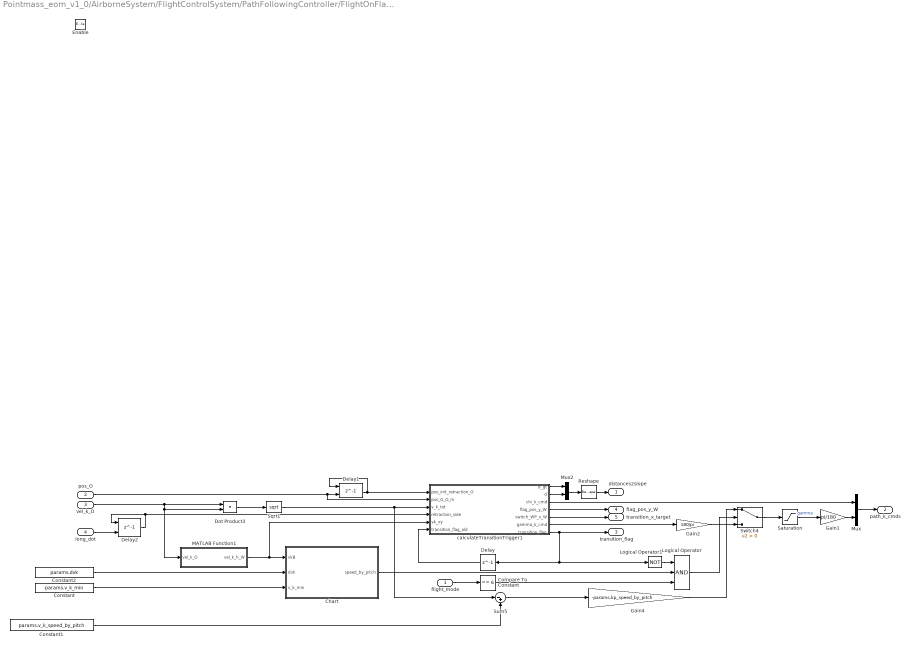
== system Pointmass_eom_v1_0/AirborneSystem/FlightControlSystem/PathFollowingController/FlightOnFlatEarth (Retraction&Loitering)/GuidanceFlatEarth/Retraction_Nav ==
  flight_mode : Inport
  pos_O : Inport  Port=2
  vel_k_O : Inport  Port=3
  long_dot : Inport  Port=4
  Enable : EnablePort  StatesWhenEnabling=reset
  Chart : Stateflow chart  TreatAsAtomicUnit=on
  Compare To Constant : simulink/Logic and Bit Operations/Compare To Constant  relop===  const=6  OutDataTypeStr=boolean
  Constant : Constant  Value=params.v_k_min
  Constant1 : Constant  Value=params.v_k_speed_by_pitch
  Constant2 : Constant  Value=params.dvk
  Delay : Delay  DelayLength=1
  Delay1 : Delay  DelayLength=1  InitialConditionSource=Input port  InitialCondition=zeros(3,1)
      settings: InputPortMap=u0,p4
  Delay2 : Delay  DelayLength=1  InitialConditionSource=Input port  InitialCondition=zeros(3,1)
      settings: InputPortMap=u0,p4
  Dot Product3 : DotProduct  InputSameDT=on  OutDataTypeStr=Inherit: Inherit via internal rule
  Gain1 : Gain  Gain=pi/180
  Gain2 : Gain  Gain=180/pi
  Gain4 : Gain  Gain=-params.kp_speed_by_pitch
  Logical Operator : Logic  Inputs=3  AllPortsSameDT=off  OutDataTypeStr=boolean
  Logical Operator1 : Logic  Operator=NOT  AllPortsSameDT=off  OutDataTypeStr=boolean
  MATLAB Function1 : MATLAB Function  TreatAsAtomicUnit=on
  Mux : Mux  Inputs=2
  Mux2 : Mux  Inputs=2
  Reshape : Reshape  OutputDimensionality=Row vector (2-D)
  Saturation : Saturate  UpperLimit=constr.gamma_max_retraction  LowerLimit=constr.gamma_min_retraction
  Sqrt1 : Sqrt  SaturateOnIntegerOverflow=on
  Sum5 : Sum  Inputs=|-+
  Switch4 : Switch  Criteria=u2 > Threshold
  calculateTransitionTrigger1 : MATLAB Function  TreatAsAtomicUnit=on
  distances2slope : Outport  VectorParamsAs1DForOutWhenUnconnected=off
  path_k_cmds : Outport  Port=2  PortDimensions=[2,1]  VectorParamsAs1DForOutWhenUnconnected=off
  transition_flag : Outport  Port=3  VectorParamsAs1DForOutWhenUnconnected=off
  flag_pos_y_W : Outport  Port=4  VectorParamsAs1DForOutWhenUnconnected=off
  transition_x_target : Outport  Port=5  VectorParamsAs1DForOutWhenUnconnected=off
  wires:
  Constant2/1 -> Chart/2(dvk)
  Constant/1 -> Chart/3(v_k_min)
  Gain2/1 -> Switch4/3
  calculateTransitionTrigger1/6(gamma_k_cmd) -> Gain2/1
  calculateTransitionTrigger1/7(transition_flag) -> transition_flag/1, Logical Operator1/1, Delay/1
  MATLAB Function1/1(vel_k_h_W) -> calculateTransitionTrigger1/5(vk_xy), Chart/1(vkB)
  Compare To Constant/1 -> Logical Operator/3
  flight_mode/1 -> Compare To Constant/1
  Chart/1(speed_by_pitch) -> Logical Operator/2
  Switch4/1 -> Saturation/1
  Gain4/1 -> Switch4/1
  Sum5/1 -> Gain4/1
  Constant1/1 -> Sum5/2
  Logical Operator/1 -> Switch4/2
  calculateTransitionTrigger1/1(d_gt) -> Mux2/1
  Mux2/1 -> Reshape/1
  calculateTransitionTrigger1/3(chi_k_cmd) -> Mux/1
  Gain1/1 -> Mux/2
  Delay1/1 -> calculateTransitionTrigger1/1(pos_init_retraction_O), Delay1/1
  Sqrt1/1 -> calculateTransitionTrigger1/3(v_k_tot), Sum5/1
  Dot Product3/1 -> Sqrt1/1
  calculateTransitionTrigger1/2(d) -> Mux2/2
  pos_O/1 -> Delay1/2, calculateTransitionTrigger1/2(pos_G_O_m)
  vel_k_O/1 -> Dot Product3/1, Dot Product3/2, MATLAB Function1/1(vel_k_O)
  Saturation/1 -> Gain1/1  "gamma"
  Mux/1 -> path_k_cmds/1
  Delay/1 -> calculateTransitionTrigger1/6(transition_flag_old)
  Logical Operator1/1 -> Logical Operator/1
  Reshape/1 -> distances2slope/1
  calculateTransitionTrigger1/4(flag_pos_y_W) -> flag_pos_y_W/1
  Delay2/1 -> calculateTransitionTrigger1/4(retraction_side), Delay2/1
  long_dot/1 -> Delay2/2
  calculateTransitionTrigger1/5(switch_WP_x_W) -> transition_x_target/1

== system Pointmass_eom_v1_0/AirborneSystem/FlightControlSystem/PathFollowingController/FlightOnSphere (Traction)/FlightPathLoopTraction/EstimatePlantResponse ==
  dphi : Inport
  alpha_rq : Inport  Port=2
  mu_k_sat : Inport  Port=3
  Ft : Inport  Port=4
  StateEstimation_Bus : Inport  Port=5
  Bus Selector : BusSelector  OutputSignals=pathangles_k,pos_G_O_m,v_k_B,airdata
  Demux : Demux  Outputs=2
  MATLAB Function : MATLAB Function  TreatAsAtomicUnit=on
  Mux : Mux  Inputs=3
  Mux4 : Mux  Inputs=2
  Selector : Selector  InputPortWidth=3  IndexOptions=Index vector (dialog)  Indices=1  OutputSizes=1
  Selector1 : Selector  InputPortWidth=3  IndexOptions=Index vector (dialog)  Indices=3  OutputSizes=1
  pathAngleRate : Outport  VectorParamsAs1DForOutWhenUnconnected=off
  wires:
  MATLAB Function/2(gamma_dot_real) -> Mux4/2
  Mux4/1 -> pathAngleRate/1
  MATLAB Function/1(chi_dot_real) -> Mux4/1
  dphi/1 -> MATLAB Function/2(dphi)
  Demux/1 -> MATLAB Function/4(chi_k)
  Demux/2 -> MATLAB Function/5(gamma_k)
  Ft/1 -> MATLAB Function/1(F_t)
  mu_k_sat/1 -> MATLAB Function/3(mu_k)
  StateEstimation_Bus/1 -> Bus Selector/1
  Bus Selector/2 -> MATLAB Function/6(pos_O)  "<pos_G_O_m>"
  Bus Selector/4 -> Selector1/1, Selector/1  "<airdata>"
  Bus Selector/3 -> MATLAB Function/7(v_k_B)  "<v_k_B>"
  Bus Selector/1 -> Demux/1  "<pathangles_k>"
  Selector/1 -> Mux/1
  Selector1/1 -> Mux/3
  alpha_rq/1 -> Mux/2
  Mux/1 -> MATLAB Function/8(airdata)

== system Pointmass_eom_v1_0/AirborneSystem/FlightControlSystem/PathFollowingController/FlightOnFlatEarth (Retraction&Loitering)/CalculateAttitudeCmds/FlightPathLoopRetraction_Aerodynamic/FlightPathLoopRetraction ==
  F_t_m : Inport
  F_t_set : Inport  Port=2
  nu_a_path : Inport  Port=3
  flightMode : Inport  Port=4
  StateEstimation_Bus : Inport  Port=5
  Bus Selector : BusSelector  OutputSignals=pos_G_O_m,pathangles_a,airdata,mu_a
  Chart : Stateflow chart  TreatAsAtomicUnit=on
  Delay : Delay  DelayLength=1  InitialConditionSource=Input port
      settings: InputPortMap=u0,p4
  Delay1 : Delay  DelayLength=1  InitialConditionSource=Input port
      settings: InputPortMap=u0,p4
  Demux : Demux  Outputs=2
  Demux1 : Demux  Outputs=2
  MATLAB Function : MATLAB Function  TreatAsAtomicUnit=on
  Transfer Fcn : TransferFcn  Numerator=[10]  Denominator=[1 10]
  inversionPathDynamics : MATLAB Function  TreatAsAtomicUnit=on
  mu_a_c : Outport  PortDimensions=1  VectorParamsAs1DForOutWhenUnconnected=off
  alpha_a_c : Outport  Port=2  PortDimensions=1  VectorParamsAs1DForOutWhenUnconnected=off
  chi_dot_real : Outport  Port=3  PortDimensions=1  VectorParamsAs1DForOutWhenUnconnected=off
  gamma_dot_real : Outport  Port=4  PortDimensions=1  VectorParamsAs1DForOutWhenUnconnected=off
  wires:
  Bus Selector/1 -> inversionPathDynamics/6(pos_O)  "<pos_G_O_m>"
  Demux1/2 -> inversionPathDynamics/8(gamma_a)
  Bus Selector/2 -> Demux1/1  "<pathangles_a>"
  Bus Selector/3 -> inversionPathDynamics/9(airdata), MATLAB Function/1(airdata)  "<airdata>"
  StateEstimation_Bus/1 -> Bus Selector/1
  Chart/1(fset) -> Transfer Fcn/1
  MATLAB Function/1(L_rq) -> Delay/2
  inversionPathDynamics/1(mu_a_c) -> Delay1/1, mu_a_c/1
  Delay1/1 -> inversionPathDynamics/1(mu_a_c_old)
  Delay/1 -> inversionPathDynamics/11(Lrq_old)
  flightMode/1 -> inversionPathDynamics/3(flightMode)
  nu_a_path/1 -> Demux/1
  Demux/2 -> inversionPathDynamics/5(nu_gamma_a)
  Demux/1 -> inversionPathDynamics/4(nu_chi_a)
  inversionPathDynamics/2(alpha_a_c) -> alpha_a_c/1
  Demux1/1 -> inversionPathDynamics/7(chi_a)
  Bus Selector/4 -> inversionPathDynamics/10(mu_a), Delay1/2  "<mu_a>"
  inversionPathDynamics/5(L_rq) -> Delay/1
  inversionPathDynamics/3(chi_dot_real) -> chi_dot_real/1
  inversionPathDynamics/4(gamma_dot_real) -> gamma_dot_real/1
  F_t_set/1 -> Chart/1(Ftset)
  F_t_m/1 -> Chart/2(Ftm)
  Transfer Fcn/1 -> inversionPathDynamics/2(f_t)

== system Pointmass_eom_v1_0/AirborneSystem/FlightControlSystem/PathFollowingController/FlightOnFlatEarth (Retraction&Loitering)/CalculateAttitudeCmds/FlightPathLoopRetraction_Aerodynamic/FlightpathReferenceModels ==
  chi_cmd : Inport
  gamma_cmd : Inport  Port=2
  gamma_hedge : Inport  Port=3
  chi_hedge : Inport  Port=4
  Mux2 : Mux  Inputs=2
  Mux3 : Mux  Inputs=2
  SecondOrderReferenceModel_course : Subsystem  mask{omega0_max=params.w0_chi_retraction_max, omega0_min=0, dynP_max=1.5312e+03, dynP_min=245.0000, zeta0=1, y_max=inf, y_min=-inf, yd_max=inf, yd_min=-inf, y2d_max=inf, y2d_min=-inf}
  SecondOrderReferenceModel_pathangle : Subsystem  mask{omega0_max=params.w0_gamma_retraction_max, omega0_min=0, dynP_max=1.5312e+03, dynP_min=245.0000, zeta0=1, y_max=inf, y_min=-inf, yd_max=inf, yd_min=-inf, y2d_max=inf, y2d_min=-inf}
  xD_ref : Outport  VectorParamsAs1DForOutWhenUnconnected=off
  x_ref : Outport  Port=2  VectorParamsAs1DForOutWhenUnconnected=off
  wires:
  gamma_hedge/1 -> SecondOrderReferenceModel_pathangle/2(hedge)
  chi_hedge/1 -> SecondOrderReferenceModel_course/2(hedge)
  gamma_cmd/1 -> SecondOrderReferenceModel_pathangle/1(y_cmd)
  chi_cmd/1 -> SecondOrderReferenceModel_course/1(y_cmd)
  Mux3/1 -> xD_ref/1
  Mux2/1 -> x_ref/1
  SecondOrderReferenceModel_course/1(y_ref) -> Mux2/1
  SecondOrderReferenceModel_pathangle/1(y_ref) -> Mux2/2
  SecondOrderReferenceModel_course/2(y_ref_dot) -> Mux3/1
  SecondOrderReferenceModel_pathangle/2(y_ref_dot) -> Mux3/2

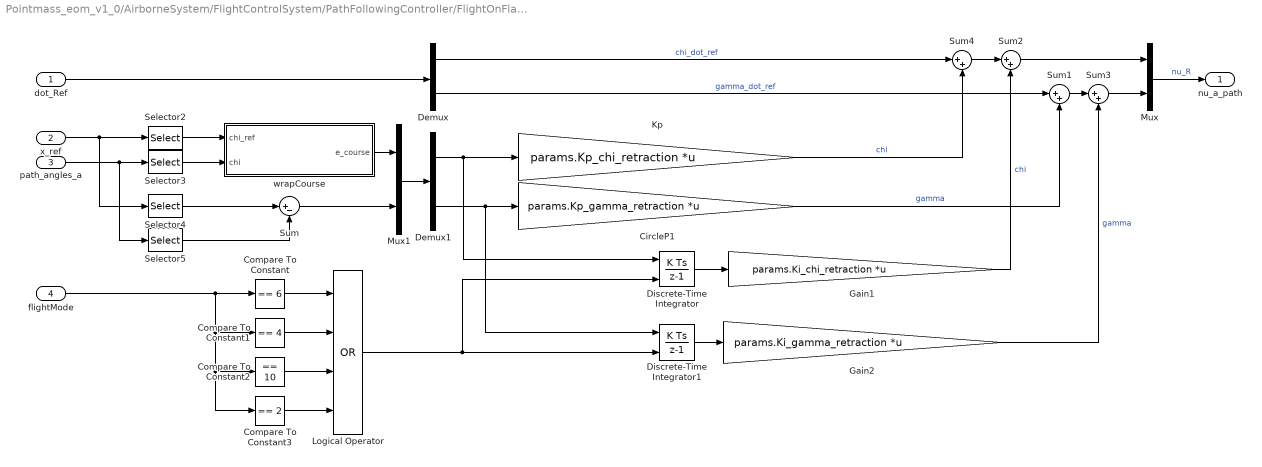
== system Pointmass_eom_v1_0/AirborneSystem/FlightControlSystem/PathFollowingController/FlightOnFlatEarth (Retraction&Loitering)/CalculateAttitudeCmds/FlightPathLoopRetraction_Aerodynamic/PIController_opt ==
  dot_Ref : Inport
  x_ref : Inport  Port=2
  path_angles_a : Inport  Port=3
  flightMode : Inport  Port=4
  CircleP1 : Gain  Gain=params.Kp_gamma_retraction  Multiplication=Matrix(K*u)
  Compare To Constant : simulink/Logic and Bit Operations/Compare To Constant  relop===  const=6  OutDataTypeStr=boolean
  Compare To Constant1 : simulink/Logic and Bit Operations/Compare To Constant  relop===  const=4  OutDataTypeStr=boolean
  Compare To Constant2 : simulink/Logic and Bit Operations/Compare To Constant  relop===  const=10  OutDataTypeStr=boolean
  Compare To Constant3 : simulink/Logic and Bit Operations/Compare To Constant  relop===  const=2  OutDataTypeStr=boolean
  Demux : Demux  Outputs=2
  Demux1 : Demux  Outputs=2
  Discrete-Time Integrator : DiscreteIntegrator  ExternalReset=either  SampleTime=-1  ICPrevOutput=DiscIntNeverNeededParam  ICPrevScaledInput=DiscIntNeverNeededParam
  Discrete-Time Integrator1 : DiscreteIntegrator  ExternalReset=either  SampleTime=-1  ICPrevOutput=DiscIntNeverNeededParam  ICPrevScaledInput=DiscIntNeverNeededParam
  Gain1 : Gain  Gain=params.Ki_chi_retraction  Multiplication=Matrix(K*u) (u vector)
  Gain2 : Gain  Gain=params.Ki_gamma_retraction  Multiplication=Matrix(K*u) (u vector)
  Kp : Gain  Gain=params.Kp_chi_retraction  Multiplication=Matrix(K*u)
  Logical Operator : Logic  Operator=OR  Inputs=4  AllPortsSameDT=off  OutDataTypeStr=boolean
  Mux : Mux  Inputs=2
  Mux1 : Mux  Inputs=2
  Selector2 : Selector  InputPortWidth=2  IndexOptions=Index vector (dialog)  Indices=1  OutputSizes=1
  Selector3 : Selector  InputPortWidth=2  IndexOptions=Index vector (dialog)  Indices=1  OutputSizes=1
  Selector4 : Selector  InputPortWidth=2  IndexOptions=Index vector (dialog)  Indices=2  OutputSizes=1
  Selector5 : Selector  InputPortWidth=2  IndexOptions=Index vector (dialog)  Indices=2  OutputSizes=1
  Sum : Sum  Inputs=|+-
  Sum{1..4} (4 alike) : Sum  Inputs=|++
  wrapCourse : MATLAB Function  TreatAsAtomicUnit=on
  nu_a_path : Outport  VectorParamsAs1DForOutWhenUnconnected=off
  wires:
  Compare To Constant3/1 -> Logical Operator/4
  Logical Operator/1 -> Discrete-Time Integrator1/2, Discrete-Time Integrator/2
  flightMode/1 -> Compare To Constant2/1, Compare To Constant3/1, Compare To Constant1/1, Compare To Constant/1
  Mux1/1 -> Demux1/1
  Mux/1 -> nu_a_path/1  "nu_R"
  dot_Ref/1 -> Demux/1
  Demux/1 -> Sum4/1  "chi_dot_ref"
  Kp/1 -> Sum4/2  "chi"
  Sum4/1 -> Sum2/1
  Demux1/1 -> Kp/1, Discrete-Time Integrator/1
  Demux/2 -> Sum1/1  "gamma_dot_ref"
  CircleP1/1 -> Sum1/2  "gamma"
  Sum1/1 -> Sum3/1
  Demux1/2 -> CircleP1/1, Discrete-Time Integrator1/1
  Compare To Constant/1 -> Logical Operator/1
  Compare To Constant1/1 -> Logical Operator/2
  Compare To Constant2/1 -> Logical Operator/3
  Discrete-Time Integrator1/1 -> Gain2/1
  path_angles_a/1 -> Selector5/1, Selector3/1
  Sum/1 -> Mux1/2
  Selector4/1 -> Sum/1
  Selector2/1 -> wrapCourse/1(chi_ref)
  x_ref/1 -> Selector4/1, Selector2/1
  wrapCourse/1(e_course) -> Mux1/1
  Gain1/1 -> Sum2/2  "chi"
  Gain2/1 -> Sum3/2  "gamma"
  Discrete-Time Integrator/1 -> Gain1/1
  Sum2/1 -> Mux/1
  Sum3/1 -> Mux/2
  Selector5/1 -> Sum/2
  Selector3/1 -> wrapCourse/2(chi)

== system Pointmass_eom_v1_0/AirborneSystem/FlightControlSystem/PathFollowingController/FlightOnFlatEarth (Retraction&Loitering)/GuidanceFlatEarth/LoiteringGuidance/Subsystem ==
  v_k_O : Inport
  h_cmd : Inport  Port=2
  h : Inport  Port=3
  Asin : Trigonometry  Operator=asin
  Divide : Product  Inputs=*/
  Dot Product : DotProduct  InputSameDT=on  OutDataTypeStr=Inherit: Inherit via internal rule
  Gain2 : Gain  Gain=-1
  Gain3 : Gain  Gain=loiterStates.kp_h
  Saturation : Saturate  UpperLimit=30*pi/180  LowerLimit=-30*pi/180
  Saturation1 : Saturate  UpperLimit=1  LowerLimit=-1
  Selector : Selector  InputPortWidth=3  IndexOptions=Index vector (dialog)  Indices=3  OutputSizes=1
  Sqrt : Sqrt  SaturateOnIntegerOverflow=on
  Sum2 : Sum  Inputs=|-+
  gamma_k_cmd : Outport  VectorParamsAs1DForOutWhenUnconnected=off
  wires:
  h_cmd/1 -> Sum2/2
  Saturation/1 -> gamma_k_cmd/1
  Selector/1 -> Gain2/1
  Gain2/1 -> Sum2/1
  Sum2/1 -> Gain3/1
  Sqrt/1 -> Divide/2
  Divide/1 -> Saturation1/1
  Dot Product/1 -> Sqrt/1
  v_k_O/1 -> Dot Product/1, Dot Product/2
  h/1 -> Selector/1
  Asin/1 -> Saturation/1
  Saturation1/1 -> Asin/1
  Gain3/1 -> Divide/1
